simulink model "AVblock"  (R2018a)
settings: Solver=FixedStepDiscrete  StartTime=0.0  StopTime=10000  FixedStep=1  MaxStep=200.0  RelTol=1e-3
libraries: model_library x4
settings Model: Creator=Arsalan  LastModifiedBy=Arsalan

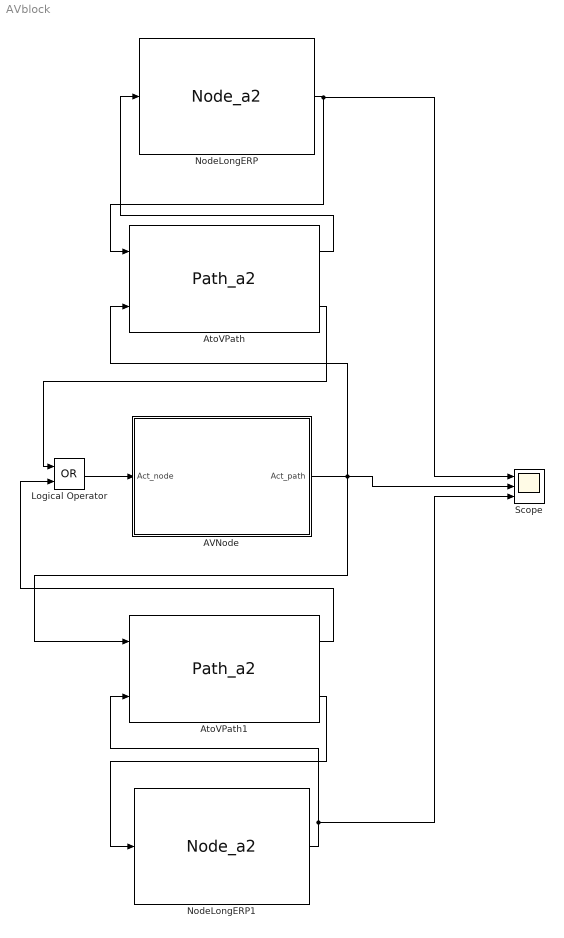
== system AVblock ==
  AVNode : Subsystem  AncestorBlock=model_library/AVNode
  AtoVPath : model_library/Path_a2
      link override Tcond_def: Value=150
  AtoVPath1 : model_library/Path_a2
      link override Tcond_def: Value=150
  Logical Operator : Logic  Operator=OR  AllPortsSameDT=off  OutDataTypeStr=boolean
  NodeLongERP : model_library/Node_a2
      link override ERP_def: Value=300
      link override Rest_def: Value=200
  NodeLongERP1 : model_library/Node_a2
      link override ERP_def: Value=300
      link override Rest_def: Value=1000
  Scope : Scope  NumInputPorts=3
  wires:
  Logical Operator/1 -> AVNode/1(Act_node)
  NodeLongERP/1 -> Scope/1, AtoVPath/1
  AtoVPath/1 -> NodeLongERP/1
  AtoVPath/2 -> Logical Operator/1
  AVNode/1(Act_path) -> Scope/2, AtoVPath1/1, AtoVPath/2
  AtoVPath1/1 -> Logical Operator/2
  AtoVPath1/2 -> NodeLongERP1/1
  NodeLongERP1/1 -> Scope/3, AtoVPath1/2

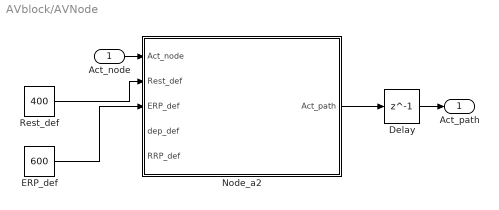
== system AVblock/AVNode ==
  Act_node : Inport
  Delay : Delay  DelayLength=1  InitialCondition=0
  ERP_def : Constant  Value=600  OutDataTypeStr=uint16
  Node_a2 : Stateflow chart  RequirementInfo="{}  %GIDa_6ee29377_7781_44c0_ad76_b00d26592997"  TreatAsAtomicUnit=on
  Rest_def : Constant  Value=400  OutDataTypeStr=uint16
  Act_path : Outport
  wires:
  Node_a2/1(Act_path) -> Delay/1
  Act_node/1 -> Node_a2/1(Act_node)
  Rest_def/1 -> Node_a2/2(Rest_def)
  ERP_def/1 -> Node_a2/3(ERP_def)
  Delay/1 -> Act_path/1

== stateflow chart AVblock/AVNode/Node_a2 ==
  state node
    settings: description=|
        | temp can be thought of a sub-mode of ERP, which only exists to make sure that act_path is high for one period.
        | 
        | In ERP, if Act_node is received, then it is ignored through that self-transition.
        | 
        | Note this doesn't model variations in cycle length because everytime it is stimulated in RRP, ERP_cur is set to ERP_def again.
    state Rest
    state RRP
    state ERP
    state temp
    (default) -> Rest : {Rest_cur=Rest_def;}
    Rest -> temp [order 3] : [Act_node==false && Rest_cur<=uint16(0)]/{Act_path=true;uptime= uint16(0);ERP_cur=ERP_def;}
    Rest -> temp [order 1] : [Act_node==true]/{Act_path=true;uptime= uint16(0);ERP_cur=ERP_def;}
    Rest -> Rest [order 2] : [Act_node==false && Rest_cur>uint16(0)]/{Rest_cur = Rest_cur - uint16(1);}
    RRP -> Rest [order 1] : [RRP_cur<=0]/{Rest_cur=Rest_def;}
    RRP -> RRP [order 2] : [Act_node==false && RRP_cur>0]/{RRP_cur=RRP_cur-uint16(1);}
    RRP -> temp [order 3] : [Act_node==true]/{Act_path=true;uptime= uint16(0);ERP_cur=ERP_def;}
    ERP -> RRP [order 1] : [ERP_cur<=uint16(0)]/{RRP_cur=RRP_def;}
    temp -> temp [order 1] : [uptime<uint16(1)]/{uptime = uptime + uint16(1);ERP_cur =ERP_cur - uint16(1);}
    temp -> ERP [order 2] : [uptime>=uint16(1)]/{Act_path=false;}
    ERP -> ERP [order 3] : [Act_node==true]
    ERP -> ERP [order 2] : {ERP_cur = ERP_cur - uint16(1);}
  data: Act_node input boolean; Act_path output boolean; Rest_cur local uint16; ERP_cur local uint16; Rest_def input uint16; ERP_def input uint16; uptime local uint16; dep_cur local uint16; dep_def input uint16; RRP_cur local uint16; RRP_def input uint16
